simulink model "FPGA_Simple_Comm_F"  (Simulink 7.6)
settings: Solver=FixedStepDiscrete  StartTime=0.0  StopTime=inf  FixedStep=0.01  MaxStep=1e-2  RelTol=1e-3
undefined symbols (not defined in the file or in its folder): Ad, Bd, Cd, Dd
libraries: simulink x10
settings Model: Creator=jordan  LastModifiedBy=jordan
settings GRTTargetCC: ExtMode=on

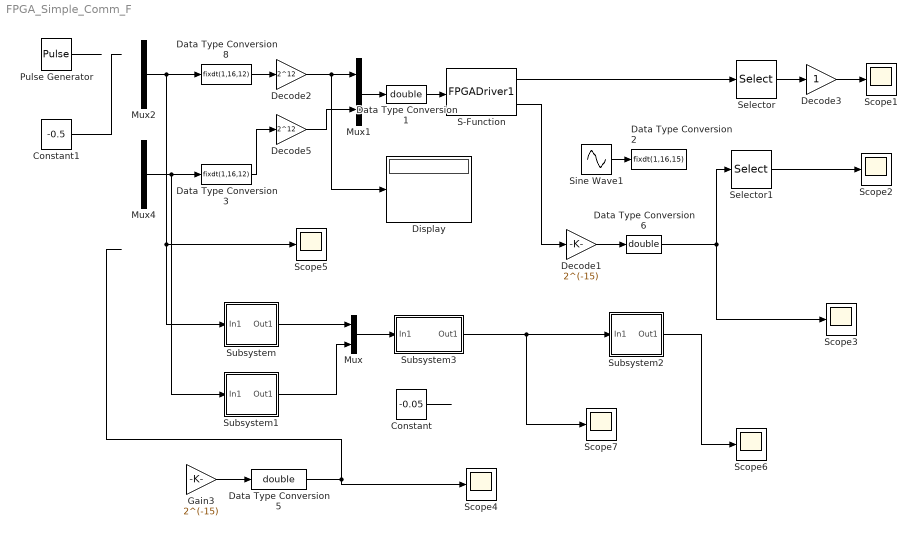
== system FPGA_Simple_Comm_F ==
  Constant : Constant  Value=-0.05
  Constant1 : Constant  Value=-0.5
  Data Type Conversion1 : DataTypeConversion  OutDataTypeStr=double
  Data Type Conversion2 : DataTypeConversion  OutDataTypeStr=fixdt(1,16,15)  SaturateOnIntegerOverflow=on
  Data Type Conversion3 : DataTypeConversion  OutDataTypeStr=fixdt(1,16,12)  SaturateOnIntegerOverflow=on
  Data Type Conversion5 : DataTypeConversion  OutDataTypeStr=double  SaturateOnIntegerOverflow=on
  Data Type Conversion6 : DataTypeConversion  OutDataTypeStr=double
  Data Type Conversion8 : DataTypeConversion  OutDataTypeStr=fixdt(1,16,12)  SaturateOnIntegerOverflow=on
  Decode1 : Gain  Gain=2^(-15)  OutDataTypeStr=fixdt(1,16,15)  SampleTime=0.01
  Decode2 : Gain  Gain=2^12  OutDataTypeStr=int16
  Decode3 : Gain  OutDataTypeStr=Inherit: Inherit via back propagation  SampleTime=0.01
  Decode5 : Gain  Gain=2^12  OutDataTypeStr=int16
  Display : Display
  Gain3 : Gain  Gain=2^(-15)  OutDataTypeStr=fixdt(1,16,15)
  Mux : Mux  Inputs=2
  Mux1 : Mux  Inputs=2
  Mux2 : Mux  Inputs=3
  Mux4 : Mux  Inputs=3
  Pulse Generator : DiscretePulseGenerator  PulseType=Time based  Amplitude=0.01  PulseWidth=50  PhaseDelay=1  SampleTime=0.01
  S-Function : S-Function  FunctionName=FPGADriver1  EnableBusSupport=off
  Scope{1..7} (7 alike) : Scope
      Scope1 settings: TimeRange=14  YMin=0  YMax=275
      Scope2 settings: TimeRange=15  YMin=-1  YMax=1  SaveName=ScopeData2
      Scope3 settings: TimeRange=4.5  YMin=0  YMax=0.0012
      Scope4 settings: TimeRange=4  YMin=0  YMax=0.2  SaveName=ScopeData3
      Scope5 settings: TimeRange=4  YMin=0  YMax=0.2  SaveName=ScopeData4
      Scope6 settings: TimeRange=4  YMin=0  YMax=0.2  SaveName=ScopeData5
      Scope7 settings: TimeRange=4  YMin=0  YMax=0.2  SaveName=ScopeData6
  Selector : Selector  InputPortWidth=4  IndexOptions=Index vector (dialog)  Indices=2  OutputSizes=1
  Selector1 : Selector  InputPortWidth=4  IndexOptions=Index vector (dialog)  Indices=1  OutputSizes=1
  Sine Wave1 : Sin  Amplitude=0.8  Frequency=2*pi  SampleTime=0.01
  Subsystem : Subsystem
  Subsystem1 : Subsystem
  Subsystem2 : Subsystem
  Subsystem3 : Subsystem
  wires:
  Sine Wave1/1 -> Data Type Conversion2/1
  Decode1/1 -> Data Type Conversion6/1
  S-Function/1 -> Selector/1
  Selector/1 -> Decode3/1
  S-Function/2 -> Decode1/1
  Decode2/1 -> Mux1/1, Display/1
  Data Type Conversion1/1 -> S-Function/1
  Decode3/1 -> Scope1/1
  Mux1/1 -> Data Type Conversion1/1
  Decode5/1 -> Mux1/2
  Mux2/1 -> Data Type Conversion8/1, Subsystem/1(In1), Scope5/1
  Mux4/1 -> Data Type Conversion3/1, Subsystem1/1(In1)
  Data Type Conversion6/1 -> Selector1/1, Scope3/1
  Data Type Conversion8/1 -> Decode2/1
  Data Type Conversion3/1 -> Decode5/1
  Subsystem/1(Out1) -> Mux/1
  Subsystem1/1(Out1) -> Mux/2
  Mux/1 -> Subsystem3/1(In1)
  Subsystem3/1(Out1) -> Subsystem2/1(In1), Scope7/1
  Subsystem2/1(Out1) -> Scope6/1
  Selector1/1 -> Scope2/1
  Gain3/1 -> Data Type Conversion5/1
  ? -> Gain3/1
  Data Type Conversion5/1 -> Scope4/1
  Constant/1 -> ?
  Pulse Generator/1 -> ?
  Constant1/1 -> ?

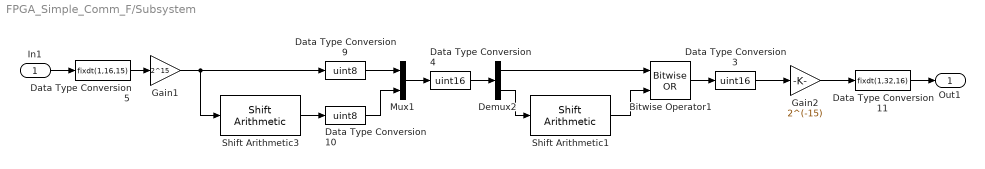
== system FPGA_Simple_Comm_F/Subsystem ==
  In1 : Inport
  Bitwise Operator1 : simulink/Logic and Bit Operations/Bitwise Operator  logicop=OR  UseBitMask=off  NumInputPorts=2  BitMask=bin2dec('11011001')  BitMaskRealWorld=Stored Integer
  Data Type Conversion10 : DataTypeConversion  OutDataTypeStr=uint8
  Data Type Conversion11 : DataTypeConversion  OutDataTypeStr=fixdt(1,32,16)
  Data Type Conversion3 : DataTypeConversion  OutDataTypeStr=uint16
  Data Type Conversion4 : DataTypeConversion  OutDataTypeStr=uint16
  Data Type Conversion5 : DataTypeConversion  OutDataTypeStr=fixdt(1,16,15)  SaturateOnIntegerOverflow=on
  Data Type Conversion9 : DataTypeConversion  OutDataTypeStr=uint8
  Demux2 : Demux  Outputs=2
  Gain1 : Gain  Gain=2^15  OutDataTypeStr=int16  SaturateOnIntegerOverflow=on
  Gain2 : Gain  Gain=2^(-15)  OutDataTypeStr=fixdt(1,16,15)
  Mux1 : Mux  Inputs=2
  Shift Arithmetic1 : simulink/Logic and Bit Operations/Shift Arithmetic  SystemSampleTime=-1  nBitShiftRight=-8  nBinPtShiftRight=0
  Shift Arithmetic3 : simulink/Logic and Bit Operations/Shift Arithmetic  SystemSampleTime=-1  nBitShiftRight=8  nBinPtShiftRight=0
  Out1 : Outport
  wires:
  Demux2/2 -> Shift Arithmetic1/1
  Demux2/1 -> Bitwise Operator1/1
  Shift Arithmetic1/1 -> Bitwise Operator1/2
  Bitwise Operator1/1 -> Data Type Conversion3/1
  Data Type Conversion4/1 -> Demux2/1
  Data Type Conversion3/1 -> Gain2/1
  Gain1/1 -> Data Type Conversion9/1, Shift Arithmetic3/1
  Shift Arithmetic3/1 -> Data Type Conversion10/1
  Data Type Conversion9/1 -> Mux1/1
  Data Type Conversion10/1 -> Mux1/2
  Mux1/1 -> Data Type Conversion4/1
  Data Type Conversion5/1 -> Gain1/1
  Gain2/1 -> Data Type Conversion11/1
  In1/1 -> Data Type Conversion5/1
  Data Type Conversion11/1 -> Out1/1

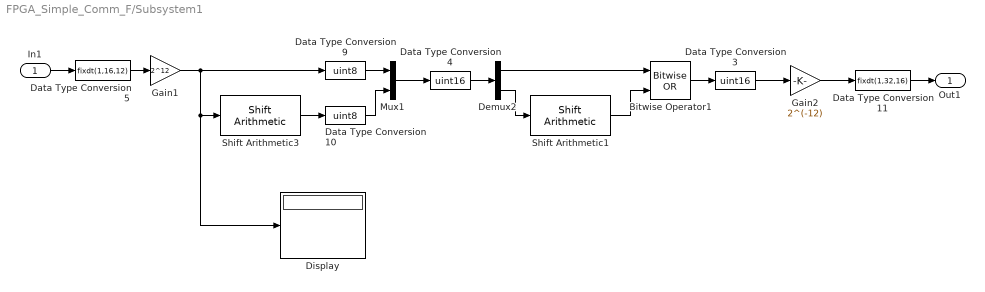
== system FPGA_Simple_Comm_F/Subsystem1 ==
  In1 : Inport
  Bitwise Operator1 : simulink/Logic and Bit Operations/Bitwise Operator  logicop=OR  UseBitMask=off  NumInputPorts=2  BitMask=bin2dec('11011001')  BitMaskRealWorld=Stored Integer
  Data Type Conversion10 : DataTypeConversion  OutDataTypeStr=uint8
  Data Type Conversion11 : DataTypeConversion  OutDataTypeStr=fixdt(1,32,16)
  Data Type Conversion3 : DataTypeConversion  OutDataTypeStr=uint16
  Data Type Conversion4 : DataTypeConversion  OutDataTypeStr=uint16
  Data Type Conversion5 : DataTypeConversion  OutDataTypeStr=fixdt(1,16,12)  SaturateOnIntegerOverflow=on
  Data Type Conversion9 : DataTypeConversion  OutDataTypeStr=uint8
  Demux2 : Demux  Outputs=2
  Display : Display
  Gain1 : Gain  Gain=2^12  OutDataTypeStr=int16  SaturateOnIntegerOverflow=on
  Gain2 : Gain  Gain=2^(-12)  OutDataTypeStr=fixdt(1,16,12)
  Mux1 : Mux  Inputs=2
  Shift Arithmetic1 : simulink/Logic and Bit Operations/Shift Arithmetic  SystemSampleTime=-1  nBitShiftRight=-8  nBinPtShiftRight=0
  Shift Arithmetic3 : simulink/Logic and Bit Operations/Shift Arithmetic  SystemSampleTime=-1  nBitShiftRight=8  nBinPtShiftRight=0
  Out1 : Outport
  wires:
  Data Type Conversion11/1 -> Out1/1
  In1/1 -> Data Type Conversion5/1
  Gain2/1 -> Data Type Conversion11/1
  Data Type Conversion5/1 -> Gain1/1
  Mux1/1 -> Data Type Conversion4/1
  Data Type Conversion10/1 -> Mux1/2
  Data Type Conversion9/1 -> Mux1/1
  Shift Arithmetic3/1 -> Data Type Conversion10/1
  Gain1/1 -> Data Type Conversion9/1, Shift Arithmetic3/1, Display/1
  Data Type Conversion3/1 -> Gain2/1
  Data Type Conversion4/1 -> Demux2/1
  Bitwise Operator1/1 -> Data Type Conversion3/1
  Shift Arithmetic1/1 -> Bitwise Operator1/2
  Demux2/1 -> Bitwise Operator1/1
  Demux2/2 -> Shift Arithmetic1/1

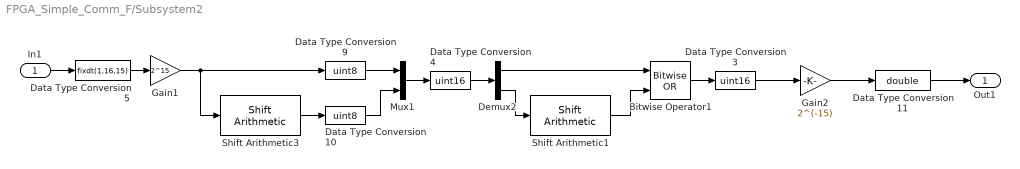
== system FPGA_Simple_Comm_F/Subsystem2 ==
  In1 : Inport
  Bitwise Operator1 : simulink/Logic and Bit Operations/Bitwise Operator  logicop=OR  UseBitMask=off  NumInputPorts=2  BitMask=bin2dec('11011001')  BitMaskRealWorld=Stored Integer
  Data Type Conversion10 : DataTypeConversion  OutDataTypeStr=uint8
  Data Type Conversion11 : DataTypeConversion  OutDataTypeStr=double
  Data Type Conversion3 : DataTypeConversion  OutDataTypeStr=uint16
  Data Type Conversion4 : DataTypeConversion  OutDataTypeStr=uint16
  Data Type Conversion5 : DataTypeConversion  OutDataTypeStr=fixdt(1,16,15)  SaturateOnIntegerOverflow=on
  Data Type Conversion9 : DataTypeConversion  OutDataTypeStr=uint8
  Demux2 : Demux  Outputs=2
  Gain1 : Gain  Gain=2^15  OutDataTypeStr=int16  SaturateOnIntegerOverflow=on
  Gain2 : Gain  Gain=2^(-15)  OutDataTypeStr=fixdt(1,16,15)
  Mux1 : Mux  Inputs=2
  Shift Arithmetic1 : simulink/Logic and Bit Operations/Shift Arithmetic  SystemSampleTime=-1  nBitShiftRight=-8  nBinPtShiftRight=0
  Shift Arithmetic3 : simulink/Logic and Bit Operations/Shift Arithmetic  SystemSampleTime=-1  nBitShiftRight=8  nBinPtShiftRight=0
  Out1 : Outport
  wires:
  Data Type Conversion11/1 -> Out1/1
  In1/1 -> Data Type Conversion5/1
  Gain2/1 -> Data Type Conversion11/1
  Data Type Conversion5/1 -> Gain1/1
  Mux1/1 -> Data Type Conversion4/1
  Data Type Conversion10/1 -> Mux1/2
  Data Type Conversion9/1 -> Mux1/1
  Shift Arithmetic3/1 -> Data Type Conversion10/1
  Gain1/1 -> Shift Arithmetic3/1, Data Type Conversion9/1
  Data Type Conversion3/1 -> Gain2/1
  Data Type Conversion4/1 -> Demux2/1
  Bitwise Operator1/1 -> Data Type Conversion3/1
  Shift Arithmetic1/1 -> Bitwise Operator1/2
  Demux2/1 -> Bitwise Operator1/1
  Demux2/2 -> Shift Arithmetic1/1

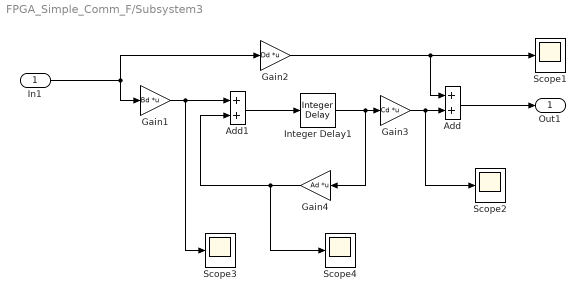
== system FPGA_Simple_Comm_F/Subsystem3 ==
  In1 : Inport
  Add : Sum  AccumDataTypeStr=fixdt(1,32,16)  OutDataTypeStr=fixdt(1,32,16)
  Add1 : Sum  AccumDataTypeStr=fixdt(1,32,16)  OutDataTypeStr=fixdt(1,32,16)
  Gain1 : Gain  Gain=Bd  Multiplication=Matrix(K*u) (u vector)  ParamDataTypeStr=fixdt(1,32,16)  OutDataTypeStr=fixdt(1,32,16)
  Gain2 : Gain  Gain=Dd  Multiplication=Matrix(K*u) (u vector)  ParamDataTypeStr=fixdt(1,32,16)  OutDataTypeStr=fixdt(1,32,16)
  Gain3 : Gain  Gain=Cd  Multiplication=Matrix(K*u) (u vector)  ParamDataTypeStr=fixdt(1,32,16)  OutDataTypeStr=fixdt(1,32,16)
  Gain4 : Gain  Gain=Ad  Multiplication=Matrix(K*u) (u vector)  ParamDataTypeStr=fixdt(1,32,16)  OutDataTypeStr=fixdt(1,32,16)
  Integer Delay1 : simulink/Discrete/Integer Delay  NumDelays=1  vinit=0.0  samptime=0.01
  Scope{1..4} (4 alike) : Scope
      Scope1 settings: TimeRange=1  YMin=-0.02  YMax=0.14  SaveName=ScopeData39
      Scope2 settings: TimeRange=1  YMin=-0.02  YMax=0.14  SaveName=ScopeData40
      Scope3 settings: TimeRange=1  YMin=-0.02  YMax=0.14  SaveName=ScopeData38
      Scope4 settings: TimeRange=1  YMin=-0.02  YMax=0.14  SaveName=ScopeData41
  Out1 : Outport
  wires:
  Integer Delay1/1 -> Gain3/1, Gain4/1
  Add1/1 -> Integer Delay1/1
  Gain1/1 -> Add1/1, Scope3/1
  Gain2/1 -> Add/1, Scope1/1
  In1/1 -> Gain2/1, Gain1/1
  Gain3/1 -> Add/2, Scope2/1
  Add/1 -> Out1/1
  Gain4/1 -> Add1/2, Scope4/1
